simulink model "Q3"  (R2025a)
settings: Solver=VariableStepAuto  StartTime=0.0  StopTime=40  RelTol=1e-3
settings Model: Creator=64892  LastModifiedBy=64892

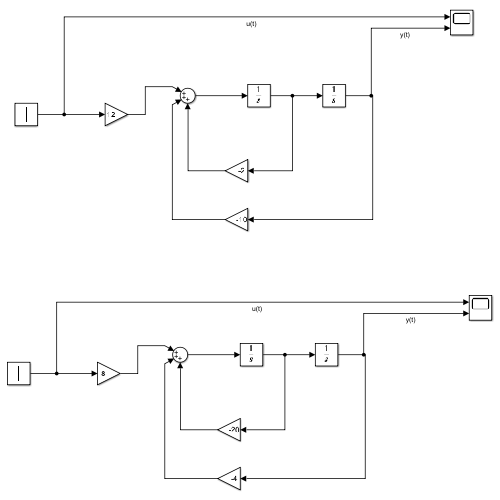
[thumbnail: Simulink's stored preview of the top-level diagram]
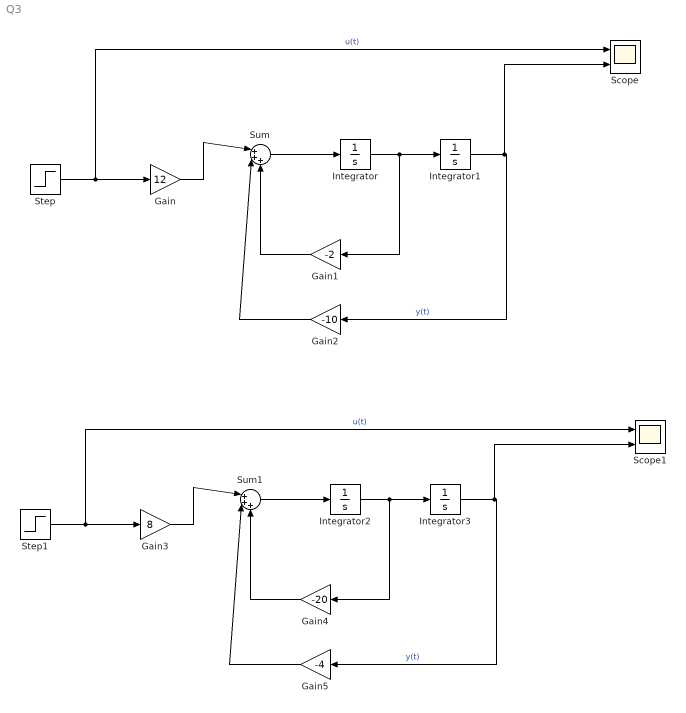
== system Q3 ==
  Gain : Gain  Gain=12
  Gain1 : Gain  Gain=-2
  Gain2 : Gain  Gain=-10
  Gain3 : Gain  Gain=8
  Gain4 : Gain  Gain=-20
  Gain5 : Gain  Gain=-4
  Integrator{,1..3} (4 alike) : Integrator
  Scope : Scope  NumInputPorts=2
      settings: ActiveDisplayYMinimum=-0.40315922551418248  ActiveDisplayYMaximum=3.6284330296276432
  Scope1 : Scope  NumInputPorts=2
      settings: ActiveDisplayYMinimum=-2.7820932800424676  ActiveDisplayYMaximum=4.45806717529581
  Step : Step  After=2  SampleTime=0
  Step1 : Step  After=2  SampleTime=0
  Sum : Sum  Inputs=|+++
  Sum1 : Sum  Inputs=|+++
  wires:
  Sum/1 -> Integrator/1
  Integrator/1 -> Gain1/1, Integrator1/1
  Integrator1/1 -> Scope/2, Gain2/1  "y(t)"
  Step/1 -> Scope/1, Gain/1  "u(t)"
  Gain/1 -> Sum/1
  Gain1/1 -> Sum/3
  Gain2/1 -> Sum/2
  Step1/1 -> Scope1/1, Gain3/1  "u(t)"
  Sum1/1 -> Integrator2/1
  Gain3/1 -> Sum1/1
  Gain4/1 -> Sum1/3
  Gain5/1 -> Sum1/2
  Integrator3/1 -> Scope1/2, Gain5/1  "y(t)"
  Integrator2/1 -> Gain4/1, Integrator3/1
